simulink model "monitor"  (R2017a)
settings: Solver=FixedStepDiscrete  StartTime=0.0  StopTime=300  FixedStep=0.01  RelTol=1e-3
PostLoadFcn:
  | bus_definitions;
StopFcn:
  | save(['data/run-', num2str(now), '.mat'], 'gpsdata', 'rawdata', 'lk_acc_state', 'ba_message', 'steering_report')
libraries: PolySyncLibrary x4, dspsigops x3
settings Model: Creator=laptopuser  LastModifiedBy=laptopuser
settings SFSimCC: SimCustomHeaderCode="#include \"MwPsTypes.hpp\""
settings SFSimCC: SimUserIncludeDirs=|
  | /home/laptopuser/Documents/MATLAB/Add-Ons/Toolboxes/PolySync/code/Inc
  | /usr/local/polysync/pdm
  | /usr/local/polysync/include
  | /usr/local/polysync/vendor/include
  | /usr/local/polysync/vendor/include/glib-2.0
  | /usr/local/polysync/include/deps
  | /usr/local/polysync/include/deps/dcps/C/SAC
  | /usr/local/polysync/include/deps/sys
  | /usr/local/polysync/plugins

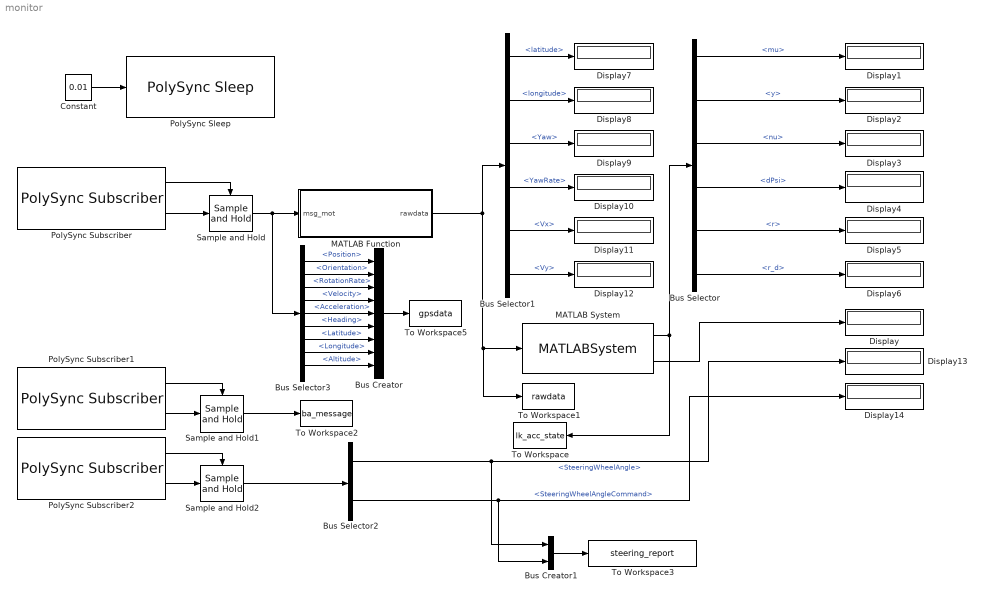
== system monitor ==
  Bus Creator : BusCreator  Inputs=9
  Bus Creator1 : BusCreator  Inputs=2
  Bus Selector : BusSelector  OutputSignals=mu,y,nu,dPsi,r,r_d
  Bus Selector1 : BusSelector  OutputSignals=latitude,longitude,Yaw,YawRate,Vx,Vy
  Bus Selector2 : BusSelector  OutputSignals=SteeringWheelAngle,SteeringWheelAngleCommand
  Bus Selector3 : BusSelector  OutputSignals=Position,Orientation,RotationRate,Velocity,Acceleration,Heading,Latitude,Longitude,Altitude
  Constant : Constant  Value=0.01
  Display{,1..14} (15 alike) : Display
  MATLAB Function : MATLAB Function  TreatAsAtomicUnit=on
  MATLAB System : MATLABSystem  System=road  lat0=42.30095833  long0=-83.69758056  h0=0  pathfile=/home/laptopuser/mkz/mcity/highway.ascii  circular=0  N_path=3  N_interp=10  dt=0.1  SimulateUsing=Code generation
      mask Type: road
      mask Display:
      | disp('road');
      | port_label('input',1,'data');
      | port_label('output',1,'lk_acc_state');
      | port_label('output',2,'road_left');
  PolySync Sleep : PolySyncLibrary/PolySync Sleep
      settings: SourceProductName=PolySync
  PolySync Subscriber : PolySyncLibrary/PolySync Subscriber  MessageType=PlatformMotionMessage  SourceGuid=0  SensorId=1  SensorType=0
      settings: SourceProductName=PolySync
  PolySync Subscriber1 : PolySyncLibrary/PolySync Subscriber  MessageType=ByteArrayMessage  SourceGuid=0  SensorId=0  SensorType=0
      settings: SourceProductName=PolySync
  PolySync Subscriber2 : PolySyncLibrary/PolySync Subscriber  MessageType=PlatformSteeringReportMessage  SourceGuid=0  SensorId=0  SensorType=0
      settings: SourceProductName=PolySync
  Sample and Hold : dspsigops/Sample and Hold  trig=Rising edge  initCond=0  latchinput=off
  Sample and Hold1 : dspsigops/Sample and Hold  trig=Rising edge  initCond=0  latchinput=off
  Sample and Hold2 : dspsigops/Sample and Hold  trig=Rising edge  initCond=0  latchinput=off
  To Workspace : ToWorkspace  VariableName=lk_acc_state  SaveFormat=Timeseries  SampleTime=-1
  To Workspace1 : ToWorkspace  VariableName=rawdata  SaveFormat=Timeseries  SampleTime=-1
  To Workspace2 : ToWorkspace  VariableName=ba_message  SaveFormat=Timeseries  SampleTime=-1
  To Workspace3 : ToWorkspace  VariableName=steering_report  SaveFormat=Timeseries  SampleTime=-1
  To Workspace5 : ToWorkspace  VariableName=gpsdata  SaveFormat=Timeseries  SampleTime=-1
  wires:
  MATLAB Function/1(rawdata) -> Bus Selector1/1, To Workspace1/1, MATLAB System/1
  MATLAB System/2 -> Display/1
  MATLAB System/1 -> Bus Selector/1, To Workspace/1
  Bus Selector/1 -> Display1/1  "<mu>"
  Bus Selector/2 -> Display2/1  "<y>"
  Bus Selector/3 -> Display3/1  "<nu>"
  Bus Selector/4 -> Display4/1  "<dPsi>"
  Bus Selector/5 -> Display5/1  "<r>"
  Bus Selector/6 -> Display6/1  "<r_d>"
  Bus Selector1/1 -> Display7/1  "<latitude>"
  Bus Selector1/2 -> Display8/1  "<longitude>"
  Bus Selector1/3 -> Display9/1  "<Yaw>"
  Bus Selector1/4 -> Display10/1  "<YawRate>"
  Bus Selector1/5 -> Display11/1  "<Vx>"
  Bus Selector1/6 -> Display12/1  "<Vy>"
  Bus Selector2/1 -> Bus Creator1/1, Display13/1  "<SteeringWheelAngle>"
  Bus Selector2/2 -> Bus Creator1/2, Display14/1  "<SteeringWheelAngleCommand>"
  Bus Selector3/1 -> Bus Creator/1  "<Position>"
  Bus Selector3/2 -> Bus Creator/2  "<Orientation>"
  Bus Selector3/3 -> Bus Creator/3  "<RotationRate>"
  Bus Selector3/4 -> Bus Creator/4  "<Velocity>"
  Bus Selector3/5 -> Bus Creator/5  "<Acceleration>"
  Bus Selector3/6 -> Bus Creator/6  "<Heading>"
  Bus Selector3/7 -> Bus Creator/7  "<Latitude>"
  Bus Selector3/8 -> Bus Creator/8  "<Longitude>"
  Bus Selector3/9 -> Bus Creator/9  "<Altitude>"
  Bus Creator/1 -> To Workspace5/1
  Bus Creator1/1 -> To Workspace3/1
  PolySync Subscriber/2 -> Sample and Hold/1
  Sample and Hold/1 -> Bus Selector3/1, MATLAB Function/1(msg_mot)
  PolySync Subscriber/1 -> Sample and Hold/Trigger
  PolySync Subscriber1/2 -> Sample and Hold1/1
  Sample and Hold1/1 -> To Workspace2/1
  PolySync Subscriber1/1 -> Sample and Hold1/Trigger
  PolySync Subscriber2/2 -> Sample and Hold2/1
  Sample and Hold2/1 -> Bus Selector2/1
  PolySync Subscriber2/1 -> Sample and Hold2/Trigger
  Constant/1 -> PolySync Sleep/1

== matlab function monitor/MATLAB Function ==
  data: msg_mot input; rawdata output Bus: DataBus
%% gps_to_rawdata:
function rawdata  = gd(msg_mot)
    rawdata = get_data(msg_mot);
